simulink model "PeripheralFluid_Insulin38"  (R2019a)
settings: Solver=VariableStepAuto  StartTime=0.0  StopTime=10.0  RelTol=1e-3
undefined symbols (not defined in the file): IPT_B, T_i_P, V_i_PF
settings Model: Creator=cgonterman  LastModifiedBy=rache
settings DataIOCC: ReturnWorkspaceOutputs=off
settings DebuggingCC: PregeneratedLibrarySubsystemCodeDiagnostic=none  ArithmeticOperatorsInVariantConditions=warning
settings SFSimCC: SimUseLocalCustomCode=off
settings RTWCC: RTWUseLocalCustomCode=off

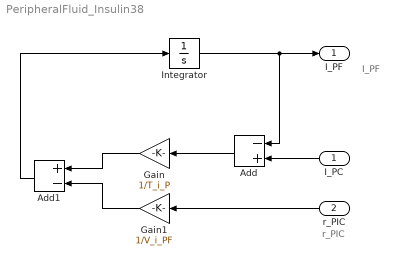
== system PeripheralFluid_Insulin38 ==
  note: I_PF
  note: r_PIC
  "I_PC " : Inport
  "r_PIC " : Inport  Port=2
  Add : Sum  Inputs=-+
  Add1 : Sum  Inputs=+-
  Gain : Gain  Gain=1/T_i_P
  Gain1 : Gain  Gain=1/V_i_PF
  Integrator : Integrator  InitialCondition=IPT_B  LimitOutput=on  LowerSaturationLimit=0
  "I_PF " : Outport
  wires:
  "r_PIC "/1 -> Gain1/1
  Gain1/1 -> Add1/2
  Gain/1 -> Add1/1
  Add/1 -> Gain/1
  "I_PC "/1 -> Add/2
  Add1/1 -> Integrator/1
  Integrator/1 -> Add/1, "I_PF "/1
